simulink model "HC_core_compensation"  (R2023b)
settings: configuration reference "slow_tsk_conf" (kept outside this file)
settings Model: DataDictionary=fmuGenerationDictionay.sldd  Creator=Veimar  LastModifiedBy=Veimar
settings ConfigSetRef: SourceName=slow_tsk_conf

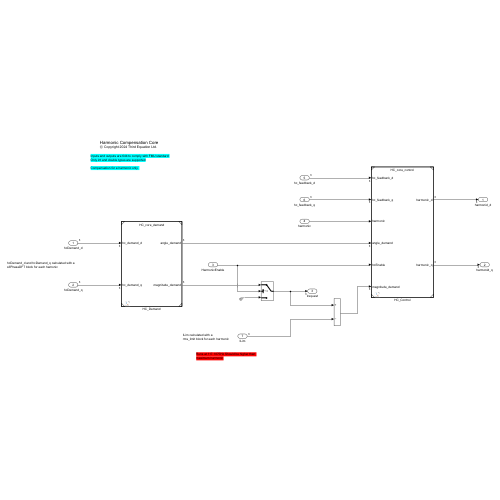
[thumbnail: Simulink's stored preview of the top-level diagram]
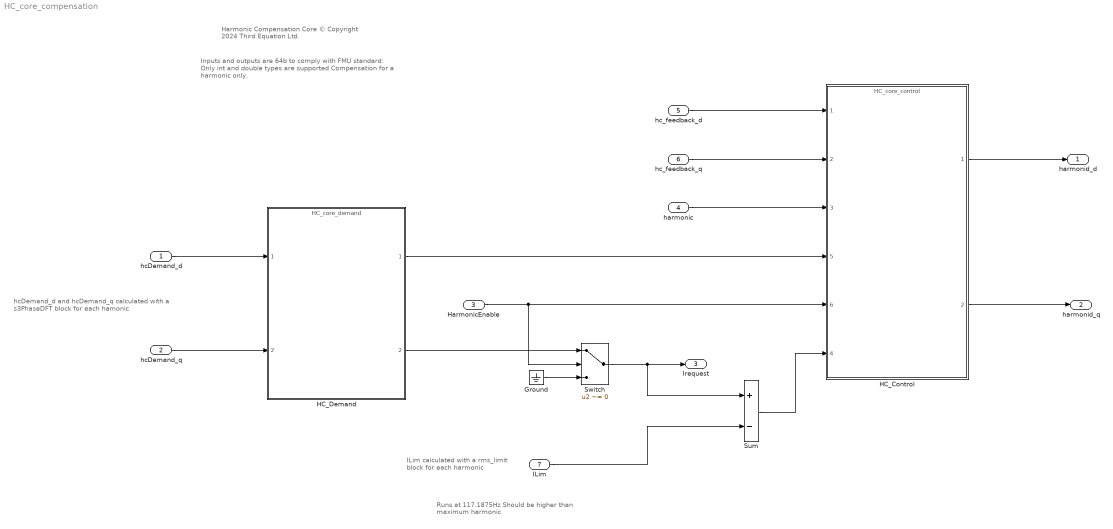
== system HC_core_compensation ==
  note: ILim calculated with a
      | rms_limit block for each harmonic
  note: hcDemand_d and hcDemand_q calculated with a
      | s3PhaseDFT block for each hamonic
  note: Harmonic Compensation Core
      | © Copyright 2024 Third Equation Ltd.
  note: Inputs and outputs are 64b to comply with FMU standard:
      | Only int and double types are supported
      |
      | Compensation for a harmonic only.
  note: Runs at 117.1875Hz Should be higher than
      | maximum harmonic
  hcDemand_d : Inport  OutDataTypeStr=single  PortDimensions=3
  hcDemand_q : Inport  Port=2  OutDataTypeStr=single  PortDimensions=3
  HarmonicEnable : Inport  Port=3  OutDataTypeStr=boolean  PortDimensions=1
  harmonic : Inport  Port=4  OutDataTypeStr=single  PortDimensions=1
  hc_feedback_d : Inport  Port=5  OutDataTypeStr=single  PortDimensions=3
  hc_feedback_q : Inport  Port=6  OutDataTypeStr=single  PortDimensions=3
  ILim : Inport  Port=7  OutDataTypeStr=single  PortDimensions=3
  Ground : Ground
  HC_Control : ModelReference  ModelNameDialog=HC_core_control.slx  SimulationMode=Normal  ModelReferenceVersion=1.59
      settings: PortSchema="{\"entries\":[{\"content\":{\"sides\":[{\"content\":{\"connectorIds\":[\"In1\",\"In2\",\"In3\",\"In5\",\"In6\",\"In4\"]},\"type\":\"ConnectorPlacement.EquallySpacedRectSide\",\"uuid\":\"85748541-43ee-4295-94aa-9804c24b54a1\"},{\"content\":{\"connectorIds\":[\"Out1\",\"Out2\"],\"side\":\"RIGHT\"},\"type\":\"ConnectorPlacement.EquallySpacedRectSide\",\"uuid\":\"50992b9a-360f-4aff-aca3-059ad107a301\"},{\"content\":{\"side\":\"TOP\"},\"type\":\"ConnectorPlacement.EquallySpacedRectSide\",\"uuid\":\"5e2b4d38-dcaf-41cd-810c-c1aa9f2a42bd\"}]},\"type\":\"ConnectorPlacement.EquallySpacedConnector\",\"uuid\":\"82905cd2-5bed-414e-bb4b-e033d05f080d\"}],\"packageUris\":[\"http://schema.mathworks.com/mf0/Connector/R2020b\"],\"version\":\"1.0\"}"
  HC_Demand : ModelReference  ModelNameDialog=HC_core_demand.slx  SimulationMode=Normal  ModelReferenceVersion=1.54
  Sum : Sum  Inputs=+-
  Switch : Switch  Criteria=u2 ~= 0  OutDataTypeStr=Inherit: Inherit via back propagation  SaturateOnIntegerOverflow=off  InputSameDT=off
  harmonid_d : Outport  OutDataTypeStr=single  PortDimensions=3
  harmonid_q : Outport  Port=2  OutDataTypeStr=single  PortDimensions=3
  Irequest : Outport  Port=3  OutDataTypeStr=single  PortDimensions=3
  wires:
  hcDemand_d/1 -> HC_Demand/1
  hcDemand_q/1 -> HC_Demand/2
  HC_Control/2 -> harmonid_q/1
  HarmonicEnable/1 -> Switch/2, HC_Control/6
  harmonic/1 -> HC_Control/3
  hc_feedback_d/1 -> HC_Control/1
  hc_feedback_q/1 -> HC_Control/2
  Sum/1 -> HC_Control/4
  Switch/1 -> Irequest/1, Sum/1
  HC_Demand/1 -> HC_Control/5
  HC_Demand/2 -> Switch/1
  Ground/1 -> Switch/3
  ILim/1 -> Sum/2
  HC_Control/1 -> harmonid_d/1
